simulink model "NoEstimationCoefficient"  (R2025b)
settings: Solver=VariableStepAuto  StartTime=0.0  StopTime=tf  FixedStep=0.001  MaxStep=tf/1e4  RelTol=1e-4  AbsTol=1e-4
values from neighbouring files (symbols this model uses):
  amplitude_disturbance = 0.3    [mainLQR.m]
  C = [1 0 0 0 ... (first row only)    [mainLQR.m]
  Qk = diag([0.1, 0.1, 0.1, 0.1])    [mainLQR.m]
  Rk = diag([10, 10])    [mainLQR.m]
  z_i = [x_i; y_i; v_i; theta_i]    [mainLQR.m]
settings Model: Creator=emanuele riva  LastModifiedBy=Utente
settings SolverCC: AutoScaleAbsTol=off  AlgebraicLoopSolver=TrustRegion
settings DataIOCC: ReturnWorkspaceOutputs=off
settings DebuggingCC: UnconnectedInputMsg=warning  UnconnectedOutputMsg=warning  UnconnectedLineMsg=warning  ArithmeticOperatorsInVariantConditions=warning
settings ModelReferenceCC: EnableRefExpFcnMdlSchedulingChecks=on
settings SFSimCC: SimUseLocalCustomCode=off  CustomCodeUndefinedFunction=UseInterfaceOnly
settings RTWCC: RTWUseLocalCustomCode=off  GPUComputeCapability=3.5  DLArmComputeVersion=19.05
settings CodeAppCC: StateflowObjectComments=on

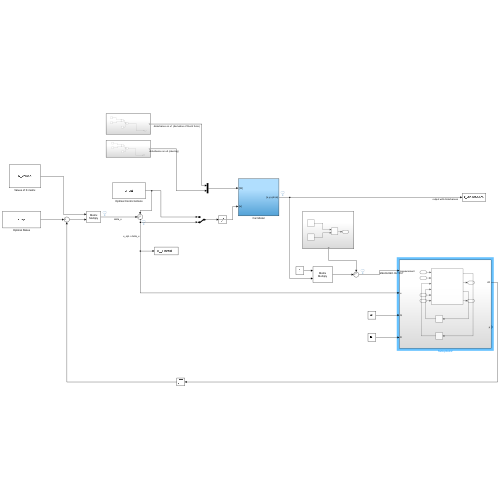
[thumbnail: Simulink's stored preview of the top-level diagram]
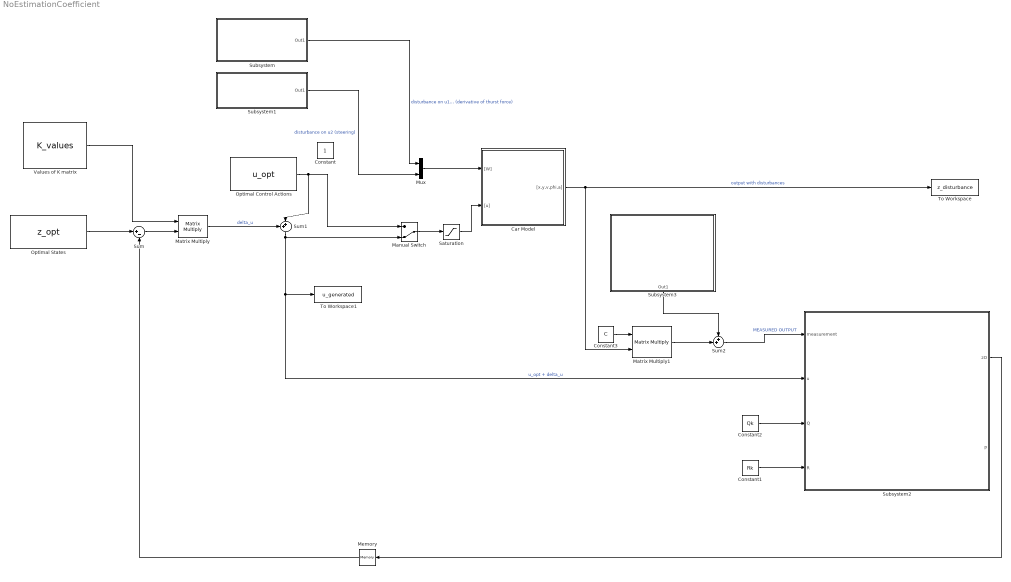
== system NoEstimationCoefficient ==
  Car Model : Subsystem
  Constant1 : Constant  Value=Rk
  Constant2 : Constant  Value=Qk
  Constant3 : Constant  Value=C
  Manual Switch : ManualSwitch  CurrentSetting=0
  Matrix Multiply : Product  Multiplication=Matrix(*)
  Matrix Multiply1 : Product  Multiplication=Matrix(*)
  Memory : Memory
  Mux : Mux  Inputs=2
  Optimal Control Actions : FromWorkspace  VariableName=u_opt
  Optimal States : FromWorkspace  VariableName=z_opt  SampleTime=-1
  Saturation : Saturate  UpperLimit=10  LowerLimit=-10
  Subsystem : Subsystem
  Subsystem1 : Subsystem
  Subsystem2 : Subsystem
  Subsystem3 : Subsystem
      settings: PortSchema="{\"entries\":[{\"content\":{\"sides\":[{\"content\":{},\"type\":\"ConnectorPlacement.EquallySpacedRectSide\",\"uuid\":\"fd3bcd80-5ad9-46ad-9bc5-a60d1158a3e8\"},{\"content\":{\"side\":\"RIGHT\"},\"type\":\"ConnectorPlacement.EquallySpacedRectSide\",\"uuid\":\"35287a45-79f5-4c20-b778-037be0434e5f\"},{\"content\":{\"side\":\"TOP\"},\"type\":\"ConnectorPlacement.EquallySpacedRectSide\",\"uuid\":\"7b704830-cfcc-4ee5-be8c-7bf24c983c1e\"},{\"content\":{\"connectorIds\":[\"Out1\"],\"side\":\"BOTTOM\"},\"type\":\"ConnectorPlacement.EquallySpacedRectSide\",\"uuid\":\"423e89fd-4d7d-4e5a-9f8e-51f01c7e5c7c\"}]},\"type\":\"ConnectorPlacement.EquallySpacedConnector\",\"uuid\":\"c34264d9-fd90-45f3-ab62-9a94c962f8b2\"}],\"packageUris\":[\"http://schema.mathworks.com/mf0/Connector/R2020b\"],\"version\":\"1.0\"}"
  Sum : Sum  Inputs=|+-
  Sum1 : Sum  Inputs=++|
  Sum2 : Sum  Inputs=++|
  To Workspace : ToWorkspace  VariableName=z_disturbance  SaveFormat=Timeseries  SampleTime=-1
  To Workspace1 : ToWorkspace  VariableName=u_generated  SaveFormat=Timeseries  SampleTime=-1
  Values of K matrix : FromWorkspace  VariableName=K_values
  Constant : Constant  IOType=siggen
  wires:
  Mux/1 -> Car Model/1("[W]")
  Subsystem/1(Out1) -> Mux/1  "disturbance on u1 (derivative of thurst force)"
  Car Model/1("[x,y,v,phi,a]") -> Matrix Multiply1/2, To Workspace/1  "output with disturbances"
  Subsystem1/1(Out1) -> Mux/2  "disturbance on u2 (steering)"
  Optimal States/1 -> Sum/1
  Sum/1 -> Matrix Multiply/2
  Values of K matrix/1 -> Matrix Multiply/1
  Matrix Multiply/1 -> Sum1/1  "delta_u"
  Sum1/1 -> Subsystem2/2(u), To Workspace1/1, Manual Switch/2  "u_opt + delta_u"
  Constant1/1 -> Subsystem2/4(R)
  Constant2/1 -> Subsystem2/3(Q)
  Sum2/1 -> Subsystem2/1(measurement)  "MEASURED OUTPUT"
  Matrix Multiply1/1 -> Sum2/2
  Subsystem3/1(Out1) -> Sum2/1
  Constant3/1 -> Matrix Multiply1/1
  Optimal Control Actions/1 -> Manual Switch/1, Sum1/2
  Subsystem2/1(zO) -> Memory/1
  Memory/1 -> Sum/2
  Manual Switch/1 -> Saturation/1
  Saturation/1 -> Car Model/2("[u]")

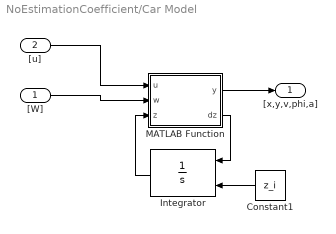
== system NoEstimationCoefficient/Car Model ==
  "[W]" : Inport
  "[u]" : Inport  Port=2
  Constant1 : Constant  Value=z_i
  Integrator : Integrator  InitialConditionSource=external
  MATLAB Function : MATLAB Function  TreatAsAtomicUnit=on
  "[x,y,v,phi,a]" : Outport
  wires:
  MATLAB Function/2(dz) -> Integrator/1
  Integrator/1 -> MATLAB Function/3(z)
  Constant1/1 -> Integrator/2
  MATLAB Function/1(y) -> "[x,y,v,phi,a]"/1
  "[u]"/1 -> MATLAB Function/1(u)
  "[W]"/1 -> MATLAB Function/2(w)

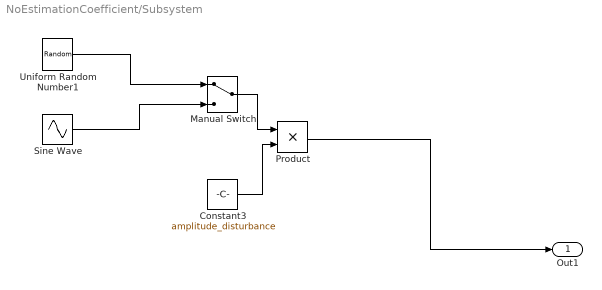
== system NoEstimationCoefficient/Subsystem ==
  Constant3 : Constant  Value=amplitude_disturbance
  Manual Switch : ManualSwitch
  Product : Product
  Sine Wave : Sin  Frequency=2*pi*100  SampleTime=0
  Uniform Random Number1 : UniformRandomNumber  SampleTime=tf/1000
  Out1 : Outport
  wires:
  Uniform Random Number1/1 -> Manual Switch/1
  Product/1 -> Out1/1
  Manual Switch/1 -> Product/1
  Sine Wave/1 -> Manual Switch/2
  Constant3/1 -> Product/2

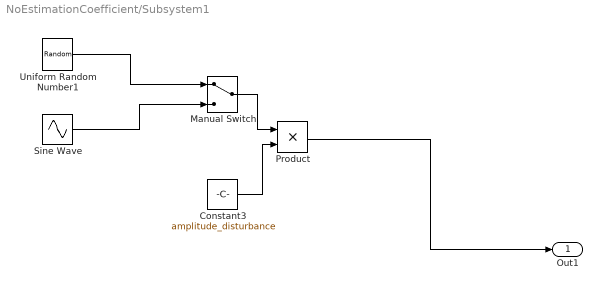
== system NoEstimationCoefficient/Subsystem1 ==
  Constant3 : Constant  Value=amplitude_disturbance
  Manual Switch : ManualSwitch
  Product : Product
  Sine Wave : Sin  Frequency=2*pi*100  SampleTime=0
  Uniform Random Number1 : UniformRandomNumber  SampleTime=tf/1000
  Out1 : Outport
  wires:
  Constant3/1 -> Product/2
  Sine Wave/1 -> Manual Switch/2
  Manual Switch/1 -> Product/1
  Product/1 -> Out1/1
  Uniform Random Number1/1 -> Manual Switch/1

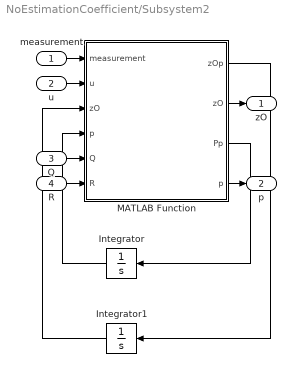
== system NoEstimationCoefficient/Subsystem2 ==
  measurement : Inport
  u : Inport  Port=2
  Q : Inport  Port=3
  R : Inport  Port=4
  Integrator : Integrator  InitialCondition=zeros(4*4,1)
  Integrator1 : Integrator  InitialCondition=z_i
  MATLAB Function : MATLAB Function  TreatAsAtomicUnit=on
  zO : Outport
  p : Outport  Port=2
  wires:
  MATLAB Function/3(Pp) -> Integrator/1
  MATLAB Function/1(zOp) -> Integrator1/1
  R/1 -> MATLAB Function/6(R)
  MATLAB Function/2(zO) -> zO/1
  Q/1 -> MATLAB Function/5(Q)
  Integrator1/1 -> MATLAB Function/3("zO ")
  Integrator/1 -> MATLAB Function/4("p ")
  measurement/1 -> MATLAB Function/1(measurement)
  u/1 -> MATLAB Function/2(u)
  MATLAB Function/4(p) -> p/1

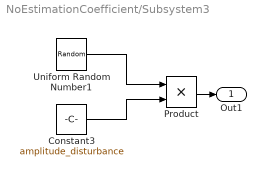
== system NoEstimationCoefficient/Subsystem3 ==
  Constant3 : Constant  Value=amplitude_disturbance
  Product : Product
  Uniform Random Number1 : UniformRandomNumber  Seed=2  SampleTime=tf/1000
  Out1 : Outport
  wires:
  Product/1 -> Out1/1
  Uniform Random Number1/1 -> Product/1
  Constant3/1 -> Product/2

== matlab function NoEstimationCoefficient/Subsystem2/MATLAB Function ==
  data: measurement input; u input; zOp output; zO input; p input; Q input; R input; zO output; Pp output; p output
function [zOp,zO,Pp,p]  = obs(measurement,u,zO,p,Q,R)

Nstates = size(zO,1);

zOp = zeros(Nstates,1);
Pp = zeros(Nstates^2,1);

% Parameters Systems:
mass = 1; %kg
Cd = 0.3; 
g = 9.81; %m/s^2
mu = 0.07;
eps = 0.1;

%% Linearization around the estimated position A,C,L

% Jacobian of the dynamics
A = [0             0            cos(zO(4))                                                                                 -zO(3)*sin(zO(4));
     0             0            sin(zO(4))                                                                                  zO(3)*cos(zO(4));
     0             0            -2*Cd*zO(3)/mass - (mu*g*sech(zO(3)/eps)^2)/eps                                              0;
     0             0            0                                                                                          0];                       

B = [0      0;
     0      0;
     1/mass 0;
     0      1];

% observation matrix

C = [1 0 0 0;
     0 1 0 0];

%% Differential Riccati Equation - Computation of the gain matrix K

% transformation vector -> matrix
P = zeros(Nstates,Nstates);
P(1:end) = p(1:end,1);

% DRE
Out = (A*P + P*A' + Q - P*C'*R^-1*C*P);

K = P*C'*R^-1;

% transformation matrix -> vector
Pp(1:end,1) = Out(1:end)';

%% State estimate


zOp(:,1) = [zO(3)*cos(zO(4));
            zO(3)*sin(zO(4));
            (u(1) - Cd*zO(3)^2 - mu*mass*g*tanh(zO(3)/eps))/mass;
            u(2)];
                                                      

zOp = zOp + K*(measurement - C*zO);

== matlab function NoEstimationCoefficient/Car Model/MATLAB Function ==
  data: u input; w input; y output; dz output; z input
function [y,dz]  = fcn(u,w,z)

mass = 1; %kg
Cd = 0.3; 
g = 9.81; %m/s^2
mu = 0.07;
eps = 0.1;

dz = zeros(4,1);

u(1) = u(1) + w(1);
u(2) = u(2) + w(2);

dz(1) = z(3)*cos(z(4));
dz(2) = z(3)*sin(z(4));
dz(3) = (u(1) - Cd*z(3)^2 - mu*mass*g*tanh(z(3)/eps))/mass;
dz(4) = u(2);
y = [z(1);z(2);z(3);z(4)];
